simulink model "plant"  (R2025b)
settings: Solver=FixedStepAuto  StartTime=0.0  StopTime=50  FixedStep=0.001  RelTol=1e-3
InitFcn:
  | rng('shuffle')
  | Cl_delta_low = rand - 1;
  | Cl_delta_high = rand + 3;
  | C0_mean = 0.001;
  | C0_bound = 0;
  | C0_low = C0_mean - C0_bound;
  | C0_high = C0_mean + C0_bound;
  | Cl_delta_delay = 0.6 * rand + 0.2;
  | C0_delay = 0.6 * rand + 0.2;
  | step_time = 0.5 * rand + 0.25;
  | step_size = (2*(rand < 0.5)-1) .* (1 + rand);
values from neighbouring files (symbols this model uses):
  idle_time = 10    [init_plant_variables.m]
libraries: aerolib6dof2 x2
settings Model: Creator=finnb  LastModifiedBy=trist

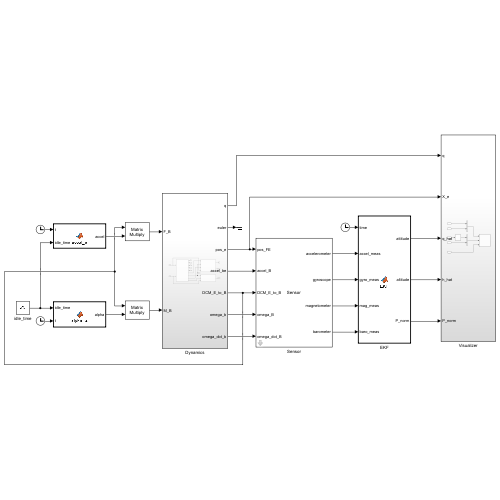
[thumbnail: Simulink's stored preview of the top-level diagram]
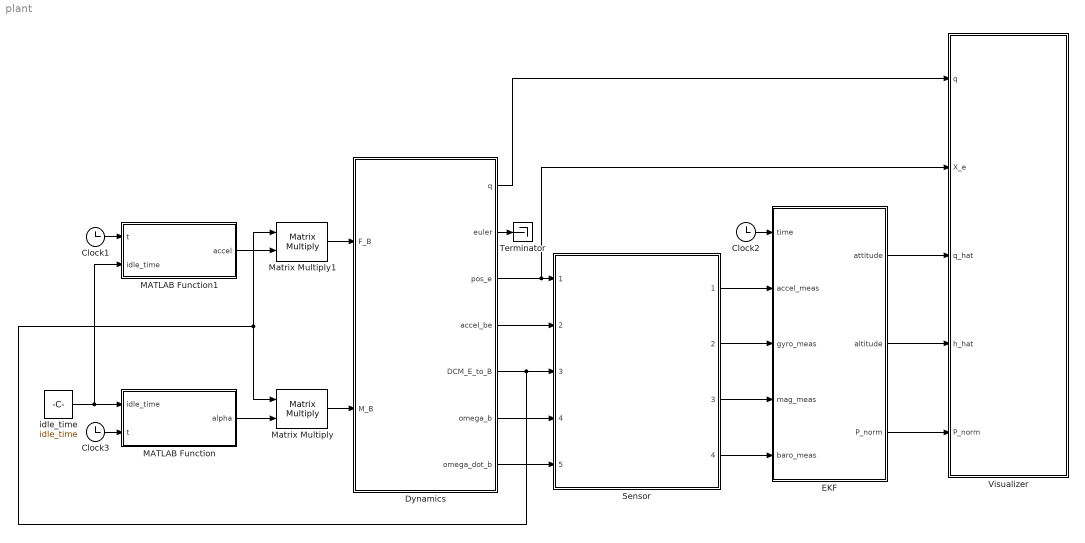
== system plant ==
  Clock1 : Clock
  Clock2 : Clock
  Clock3 : Clock
  Dynamics : Subsystem
  EKF : MATLAB Function  TreatAsAtomicUnit=on
  MATLAB Function : MATLAB Function  TreatAsAtomicUnit=on
  MATLAB Function1 : MATLAB Function  TreatAsAtomicUnit=on
  Matrix Multiply : Product  Multiplication=Matrix(*)
  Matrix Multiply1 : Product  Multiplication=Matrix(*)
  Sensor : Subsystem  ReferencedSubsystem=Sensor  Parameter22=0  Parameter23=0  noise_accel=[1,1,1]*6.7e-8  bias_accel=[1,1,1]*0.1  scale_accel=[1 0 0; 0 1 0; 0 0 1]  lim_accel=39.2  noise_gyro=[1,1,1]*6.9e-9  bias_gyro=[1,1,1]*pi/180  scale_gyro=[1 0 0; 0 1 0; 0 0 1]  lim_gyro=34.9  noise_mag=[1,1,1]*3.6e-8  bias_mag=[1,1,1]*0.02  scale_mag=[1 0 0; 0 1 0; 0 0 1]  limit_mag=13  noise_pres=0.004  bias_pres=50  scale_pres=1  limit_pres=[30000 125000]  Ssi=[1 0 0; 0 1 0; 0 0 1]  Lsi=[0 0 0]  lon=-80.5204  lat=43.4643  year=2025  samplingrate=0.001
  Terminator : Terminator
  Visualizer : Subsystem
  idle_time : Constant  Value=idle_time
  wires:
  Matrix Multiply/1 -> Dynamics/2(M_B)
  Dynamics/5(DCM_E_to_B) -> Matrix Multiply1/1, Matrix Multiply/1, Sensor/3
  Matrix Multiply1/1 -> Dynamics/1(F_B)
  MATLAB Function1/1(accel) -> Matrix Multiply1/2
  Clock1/1 -> MATLAB Function1/1(t)
  MATLAB Function/1(alpha) -> Matrix Multiply/2
  Sensor/1 -> EKF/2(accel_meas)
  Sensor/2 -> EKF/3(gyro_meas)
  Sensor/3 -> EKF/4(mag_meas)
  Sensor/4 -> EKF/5(baro_meas)
  idle_time/1 -> MATLAB Function/1(idle_time), MATLAB Function1/2(idle_time)
  Clock2/1 -> EKF/1(time)
  Dynamics/3(pos_e) -> Visualizer/2(X_e), Sensor/1
  Dynamics/4(accel_be) -> Sensor/2
  Dynamics/6(omega_b) -> Sensor/4
  Dynamics/7(omega_dot_b) -> Sensor/5
  Dynamics/2(euler) -> Terminator/1
  Dynamics/1(q) -> Visualizer/1(q)
  EKF/1(attitude) -> Visualizer/3(q_hat)
  EKF/2(altitude) -> Visualizer/4(h_hat)
  EKF/3(P_norm) -> Visualizer/5(P_norm)
  Clock3/1 -> MATLAB Function/2(t)

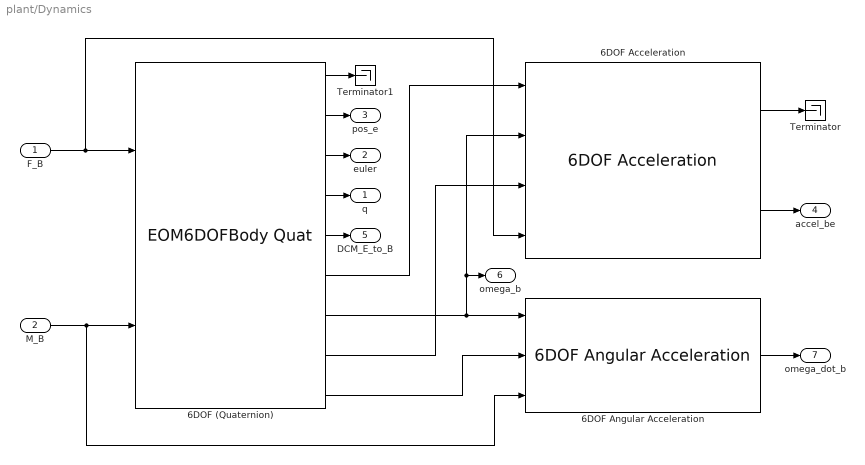
== system plant/Dynamics ==
  F_B : Inport
  M_B : Inport  Port=2
  6DOF (Quaternion) : EOM6DOFBodyQuat  mass_flag=on
  6DOF Acceleration : aerolib6dof2/6DOF Acceleration  units=Metric (MKS)  mtype=Fixed  vre_flag=off
  6DOF Angular Acceleration : aerolib6dof2/6DOF Angular Acceleration  units=Metric (MKS)  mtype=Fixed
  Terminator : Terminator
  Terminator1 : Terminator
  q : Outport
  euler : Outport  Port=2
  pos_e : Outport  Port=3
  accel_be : Outport  Port=4
  DCM_E_to_B : Outport  Port=5
  omega_b : Outport  Port=6
  omega_dot_b : Outport  Port=7
  wires:
  F_B/1 -> 6DOF Acceleration/4, 6DOF (Quaternion)/1
  M_B/1 -> 6DOF Angular Acceleration/3, 6DOF (Quaternion)/2
  6DOF (Quaternion)/9 -> 6DOF Angular Acceleration/2
  6DOF (Quaternion)/8 -> 6DOF Acceleration/3
  6DOF (Quaternion)/7 -> 6DOF Acceleration/2, omega_b/1, 6DOF Angular Acceleration/1
  6DOF (Quaternion)/6 -> 6DOF Acceleration/1
  6DOF (Quaternion)/2 -> pos_e/1
  6DOF Acceleration/2 -> accel_be/1
  6DOF Angular Acceleration/1 -> omega_dot_b/1
  6DOF Acceleration/1 -> Terminator/1
  6DOF (Quaternion)/5 -> DCM_E_to_B/1
  6DOF (Quaternion)/4 -> q/1
  6DOF (Quaternion)/3 -> euler/1
  6DOF (Quaternion)/1 -> Terminator1/1

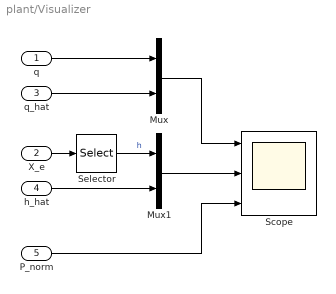
== system plant/Visualizer ==
  q : Inport
  X_e : Inport  Port=2
  q_hat : Inport  Port=3
  h_hat : Inport  Port=4
  P_norm : Inport  Port=5
  Mux : Mux  Inputs=2
  Mux1 : Mux  Inputs=2
  Scope : Scope  NumInputPorts=3
      settings: ActiveDisplayYMinimum=-1.2452023842361069  ActiveDisplayYMaximum=1.2494669315817897
  Selector : Selector  InputPortWidth=3  IndexOptions=Index vector (dialog)  Indices=3  OutputSizes=1
  wires:
  Mux/1 -> Scope/1
  q_hat/1 -> Mux/2
  q/1 -> Mux/1
  X_e/1 -> Selector/1
  Mux1/1 -> Scope/2
  h_hat/1 -> Mux1/2
  Selector/1 -> Mux1/1  "h"
  P_norm/1 -> Scope/3

== matlab function plant/MATLAB Function1 ==
  settings: updateMethod=DISCRETE  sampleTime=0.01
  data: t input; accel output; idle_time input
function accel = accel_e(t, idle_time)
%#codegen
% 3-axis acceleration excitation: sine + Gaussian noise

accel = [0; 0; 0];


if t >= idle_time
    A = [0.5; 0.5; 0.5];      % amplitudes
    f = [0.25; 0.25; 0.25];  % frequencies (Hz)
    phi = [0; 0; 0];         % phases (rad)
    
    sigma = 0.1;             % noise std dev
    
    accel = [0; 0; 0]; %A .* sin(2*pi*f*t + phi) + sigma * randn(3,1);
end

== matlab function plant/MATLAB Function ==
  settings: updateMethod=DISCRETE  sampleTime=0.01
  data: idle_time input; t input; alpha output
function alpha = alpha_e(idle_time, t)
%#codegen
% 3-axis excitation: sine + Gaussian noise

alpha = [0;0;0];

if t > idle_time
    A = [0.3; 0.2; 0.1];     % amplitudes
    f = [0.25; 0.15; 0.45]; % frequencies (Hz)
    phi = [0; 0; 0];        % phases (rad)
    
    sigma = 0;            % noise std dev
    
    alpha = A .* sin(2*pi*f*t + phi) + sigma * randn(3,1);
end

== matlab function plant/EKF ==
  settings: updateMethod=DISCRETE  sampleTime=0.01
  data: time input; accel_meas input; attitude output; altitude output; gyro_meas input; mag_meas input; baro_meas input; P_norm output
function [attitude, altitude, P_norm] = EKF(time, accel_meas, gyro_meas, mag_meas, baro_meas)
    
    persistent k
    if isempty(k)
        k = 0;
    end

    accel.meas = accel_meas;
    gyro.meas = gyro_meas;
    mag.meas = mag_meas;
    baro.meas = baro_meas;

    accel.status = mod(k, 10) == 0;    % 100 Hz
    gyro.status = mod(k, 10) == 0;    % 100 Hz
    mag.status = mod(k, 50) == 23;   % 20 Hz
    baro.status = mod(k, 40) == 7;    % 25 Hz

    k = mod(k + 1, 200);    % lcm(10, 40, 50)

    [attitude, altitude, P_norm] = filter_caller(time, accel, gyro, mag, baro);
end
